simulink subsystem "EncoderDistancia"  (R2023b)
settings: Solver=VariableStepAuto  StartTime=0.0  StopTime=10.0  RelTol=1e-3
libraries: arduinosensorlib x2
settings Model: Creator=chaya  LastModifiedBy=chaya

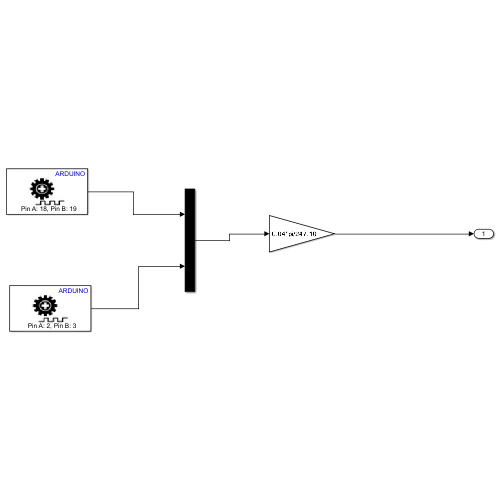
[thumbnail: Simulink's stored preview of the top-level diagram]
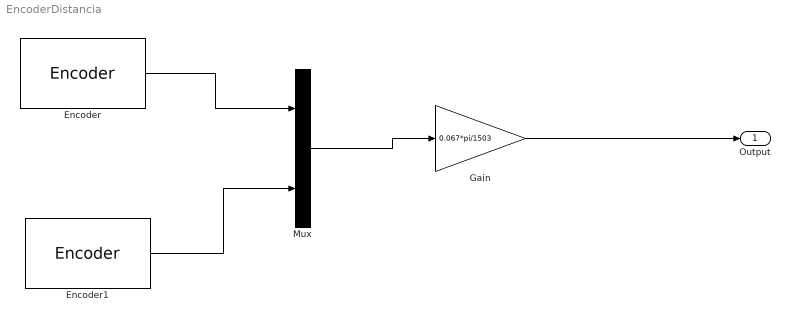
== system EncoderDistancia ==
  Encoder : arduinosensorlib/Encoder  InputA=18  InputB=19  Mode=No reset  SampleTime=-1
  Encoder1 : arduinosensorlib/Encoder  InputA=2  InputB=3  Mode=No reset  SampleTime=-1
  Gain : Gain  Gain=0.067*pi/1503
  Mux : Mux  Inputs=2
  Output : Outport
  wires:
  Encoder/1 -> Mux/1
  Encoder1/1 -> Mux/2
  Mux/1 -> Gain/1
  Gain/1 -> Output/1
